simulink model "aae564hw02p78"  (R2021a)
settings: Solver=VariableStepAuto  StartTime=0.0  StopTime=10.0  MaxStep=1e-6  RelTol=1e-6
settings Model: Creator=Joseph  LastModifiedBy=Joseph

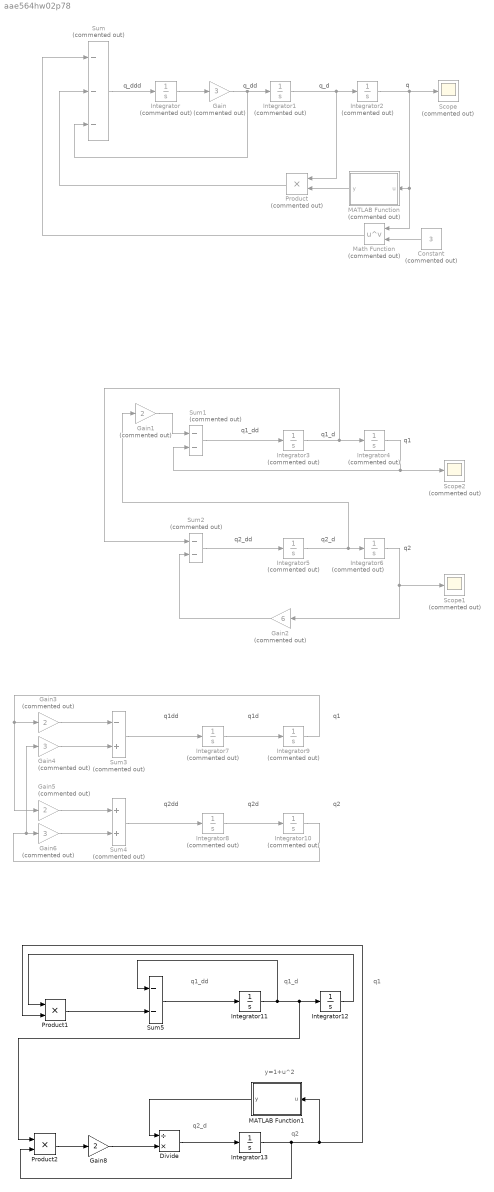
== system aae564hw02p78 ==
  note: y=1+u^2
  note: q1
  note: q1_d
  note: q2
  note: q1_dd
  note: q2
  note: q2d
  note: q2dd
  note: q1
  note: q1d
  note: q1dd
  note: q2
  note: q1
  note: q1_d
  note: q1_dd
  note: q
  note: q_d
  note: q_dd
  note: q_ddd
  note: q2_d
  note: q2_dd
  note: q2_d
  Constant : Constant  Commented=on  Value=3
  Divide : Product  Inputs=/*
  Gain : Gain  Commented=on  Gain=3
  Gain1 : Gain  Commented=on  Gain=2
  Gain2 : Gain  Commented=on  Gain=6
  Gain3 : Gain  Commented=on  Gain=2
  Gain4 : Gain  Commented=on  Gain=3
  Gain5 : Gain  Commented=on  Gain=2
  Gain6 : Gain  Commented=on  Gain=3
  Gain8 : Gain  Gain=2
  Integrator{,2..10} (10 alike) : Integrator  Commented=on
  Integrator1 : Integrator  Commented=on  InitialCondition=1
  Integrator11 : Integrator
  Integrator12 : Integrator
  Integrator13 : Integrator
  MATLAB Function : MATLAB Function  Commented=on  TreatAsAtomicUnit=on
  MATLAB Function1 : MATLAB Function  TreatAsAtomicUnit=on
  Math Function : Math  Commented=on  Operator=pow  SaturateOnIntegerOverflow=on
  Product : Product  Commented=on
  Product1 : Product
  Product2 : Product
  Scope : Scope  Commented=on
  Scope1 : Scope  Commented=on
  Scope2 : Scope  Commented=on
  Sum : Sum  Commented=on  Inputs=---
  Sum1 : Sum  Commented=on  Inputs=--
  Sum2 : Sum  Commented=on  Inputs=--
  Sum3 : Sum  Commented=on  Inputs=-+
  Sum4 : Sum  Commented=on
  Sum5 : Sum  Inputs=--
  wires:
  Integrator2/1 -> Scope/1, Math Function/1, MATLAB Function/1(u)
  Integrator1/1 -> Product/1, Integrator2/1
  Integrator/1 -> Gain/1
  Gain/1 -> Sum/3, Integrator1/1
  Sum/1 -> Integrator/1
  MATLAB Function/1(y) -> Product/2
  Product/1 -> Sum/2
  Math Function/1 -> Sum/1
  Constant/1 -> Math Function/2
  Integrator3/1 -> Sum2/1, Integrator4/1
  Gain1/1 -> Sum1/1
  Sum1/1 -> Integrator3/1
  Sum2/1 -> Integrator5/1
  Integrator4/1 -> Scope2/1, Sum1/2
  Integrator6/1 -> Gain2/1, Scope1/1
  Integrator5/1 -> Gain1/1, Integrator6/1
  Gain2/1 -> Sum2/2
  Integrator7/1 -> Integrator9/1
  Integrator8/1 -> Integrator10/1
  Sum4/1 -> Integrator8/1
  Sum3/1 -> Integrator7/1
  Gain5/1 -> Sum4/1
  Gain6/1 -> Sum4/2
  Gain4/1 -> Sum3/2
  Gain3/1 -> Sum3/1
  Integrator9/1 -> Gain3/1, Gain5/1
  Integrator10/1 -> Gain4/1, Gain6/1
  Sum5/1 -> Integrator11/1
  Integrator11/1 -> Sum5/1, Product2/1, Integrator12/1
  Integrator13/1 -> Product2/2, MATLAB Function1/1(u), Product1/2
  Product1/1 -> Sum5/2
  Integrator12/1 -> Product1/1
  Product2/1 -> Gain8/1
  Gain8/1 -> Divide/2
  MATLAB Function1/1(y) -> Divide/1
  Divide/1 -> Integrator13/1

== matlab function aae564hw02p78/MATLAB Function ==
  data: u input; y output
function y = fcn(u)

y = sin(u);

== matlab function aae564hw02p78/MATLAB Function1 ==
  data: u input; y output
function y = fcn(u)

y = 1+u^2;
